simulink subsystem "ControlSystem"  (R2023a)
settings: Solver=VariableStepAuto  StartTime=0.0  StopTime=10.0  RelTol=1e-3
settings Model: Creator=Alla  LastModifiedBy=Alla

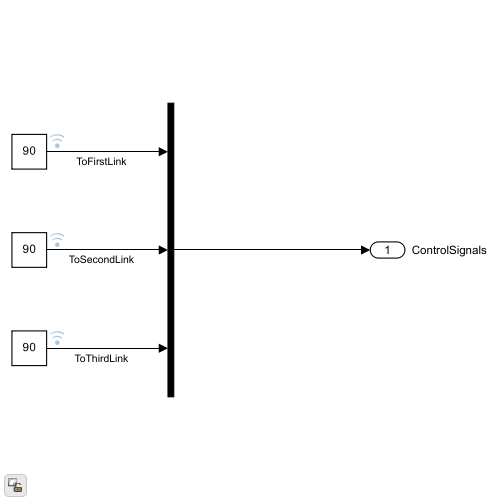
[thumbnail: Simulink's stored preview of the top-level diagram]
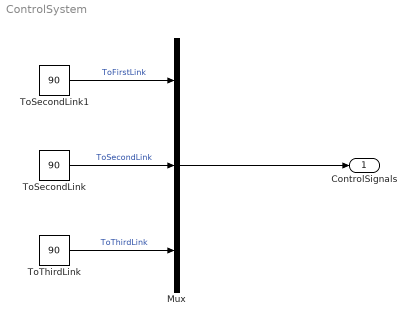
== system ControlSystem ==
  Mux : Mux  Inputs=3
  ToSecondLink : Constant  Value=90
  ToSecondLink1 : Constant  Value=90
  ToThirdLink : Constant  Value=90
  ControlSignals : Outport
  wires:
  Mux/1 -> ControlSignals/1
  ToSecondLink/1 -> Mux/2  "ToSecondLink"
  ToSecondLink1/1 -> Mux/1  "ToFirstLink"
  ToThirdLink/1 -> Mux/3  "ToThirdLink"
